simulink model "prodinvsys_ol"  (R2021b)
settings: Solver=ode15s  StartTime=0.0  StopTime=10.0  RelTol=1e-3  AbsTol=1e-6
values from neighbouring files (symbols this model uses):
  dchange = [60, 150]    [run_sim_ol.m]    (also in run_sim_spec.m = sim_spec.dchange; singlenodescm2022.m = input('Enter the demand change [2000 units]: '))
  rchange = [10, 1000]    [run_sim_ol.m]    (also in run_sim_spec.m = sim_spec.rchange; singlenodescm2022.m = input('Enter the inventory setpoint [20000 units]: '))
  thetaf = 20    [run_sim_ol.m]
  thetap = 10    [run_sim_ol.m]    (also in run_sim_spec.m = sim_spec.thetap; singlenodescm2022.m = input('Enter the production lead time (thetap) [10 time unit)
  thetas = 2    [run_sim_ol.m]    (also in run_sim_spec.m = sim_spec.thetas; singlenodescm2022.m = input('Enter the supply stream delivery time (thetad) [2 tim)
  Ts = 1    [run_sim_ol.m]
  vard = [85, 1000]    [run_sim_ol.m]    (also in run_sim_spec.m = sim_spec.vard; singlenodescm2022.m = input('Enter the unforecasted demand variance (vard) [1000]:)
settings Model: Creator=derivera  LastModifiedBy=billtubbs
settings SolverCC: AutoScaleAbsTol=off  AlgebraicLoopSolver=TrustRegion
settings DataIOCC: SaveFormat=Array  SignalLoggingSaveFormat=ModelDataLogs  ReturnWorkspaceOutputs=off
settings OptimizationCC: BooleanDataType=off  LifeSpan=inf
settings DebuggingCC: SaveWithParameterizedLinksMsg=none  UnderspecifiedInitializationDetection=Classic  MergeDetectMultiDrivingBlocksExec=none  SignalResolutionControl=TryResolveAllWithWarning  MultiTaskDSMMsg=warning  MultiTaskCondExecSysMsg=none  SFUnexpectedBacktrackingDiag=warning  SFNoUnconditionalDefaultTransitionDiag=warning  SFExecutionAtInitializationDiag=none  SFMachineParentedDataDiag=warning  ArithmeticOperatorsInVariantConditions=warning
settings HardwareCC: ProdBitPerPointer=32  ProdBitPerSizeT=32  ProdBitPerPtrDiffT=32  ProdLargestAtomicFloat=None  ProdIntDivRoundTo=Undefined  ProdEndianess=Unspecified  ProdWordSize=32  ProdHWDeviceType=32-bit Generic  TargetUnknown=on
settings ModelReferenceCC: PropagateSignalLabelsOutOfModel=off
settings SFSimCC: SimUseLocalCustomCode=off  CustomCodeUndefinedFunction=UseInterfaceOnly
settings RTWCC: RTWUseLocalCustomCode=off
settings CodeAppCC: StateflowObjectComments=on
settings GRTTargetCC: TargetLangStandard=C89/C90 (ANSI)  CombineOutputUpdateFcns=off  GRTInterface=on
settings ConfigComp: CovMetricSettings=dw  CovSaveCumulativeToWorkspaceVar=on  CovSaveSingleToWorkspaceVar=on  CovExternalEMLEnable=off  CovSFcnEnable=off

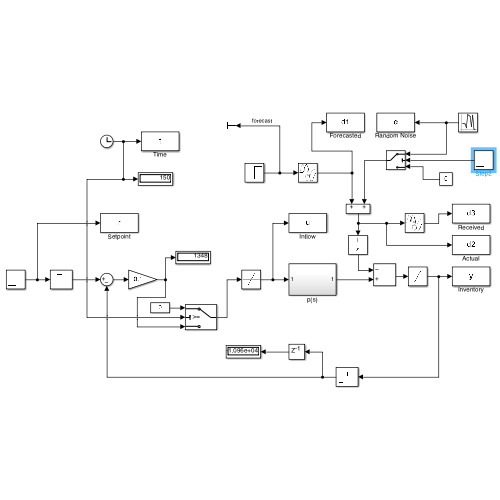
[thumbnail: Simulink's stored preview of the top-level diagram]
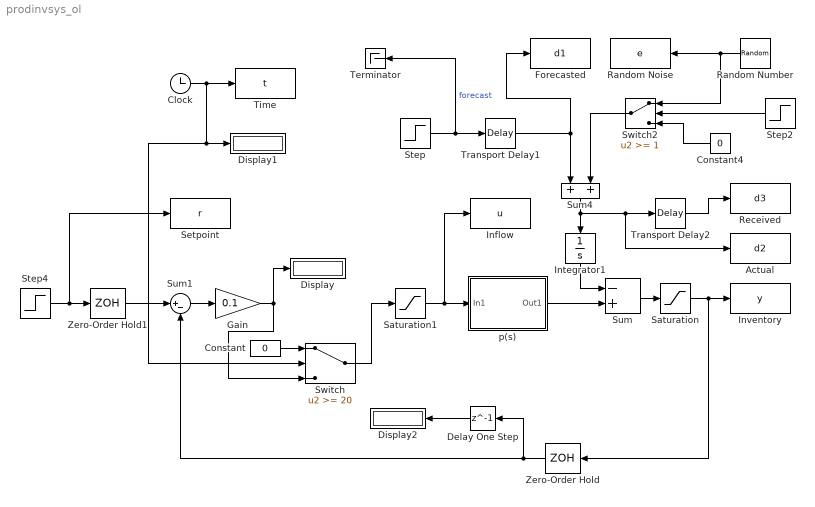
== system prodinvsys_ol ==
  Actual : ToWorkspace  VariableName=d2  SampleTime=Ts
  Clock : Clock
  Constant : Constant  Value=0
  Constant4 : Constant  Value=0
  Delay One Step : Delay  DelayLength=1
  Display : Display
  Display1 : Display
  Display2 : Display
  Forecasted : ToWorkspace  VariableName=d1  SampleTime=Ts
  Gain : Gain  Gain=0.1
  Inflow : ToWorkspace  VariableName=u  SampleTime=Ts
  Integrator1 : Integrator
  Inventory : ToWorkspace  VariableName=y  SampleTime=Ts
  Random Number : RandomNumber  Variance=vard(2)  SampleTime=1
  Random Noise : ToWorkspace  VariableName=e  SampleTime=Ts
  Received : ToWorkspace  VariableName=d3  SampleTime=Ts
  Saturation : Saturate  UpperLimit=inf  LowerLimit=-inf
  Saturation1 : Saturate  UpperLimit=inf  LowerLimit=-inf
  Setpoint : ToWorkspace  VariableName=r  SampleTime=Ts
  Step : Step  Time=dchange(1) - thetaf  After=dchange(2)  SampleTime=0
  Step2 : Step  Time=vard(1)  SampleTime=0
  Step4 : Step  Time=rchange(1)  After=rchange(2)  SampleTime=0
  Sum : Sum  Inputs=-+  InputSameDT=on  SaturateOnIntegerOverflow=on  OutDataTypeStr=Inherit: Same as first input
  Sum1 : Sum  Inputs=|+-
  Sum4 : Sum  InputSameDT=on  SaturateOnIntegerOverflow=on  OutDataTypeStr=Inherit: Same as first input
  Switch : Switch  Threshold=20
  Switch2 : Switch  Threshold=1  SaturateOnIntegerOverflow=on  InputSameDT=on
  Terminator : Terminator
  Time : ToWorkspace  VariableName=t  SampleTime=Ts
  Transport Delay1 : TransportDelay  DelayTime=thetaf
  Transport Delay2 : TransportDelay  DelayTime=thetas
  Zero-Order Hold : ZeroOrderHold  SampleTime=10
  Zero-Order Hold1 : ZeroOrderHold  SampleTime=10
  p(s) : Subsystem
  wires:
  p(s)/1(Out1) -> Sum/2
  Integrator1/1 -> Sum/1
  Sum/1 -> Saturation/1
  Saturation/1 -> Zero-Order Hold/1, Inventory/1
  Saturation1/1 -> Inflow/1, p(s)/1(In1)
  Step/1 -> Terminator/1, Transport Delay1/1  "forecast"
  Transport Delay2/1 -> Received/1
  Sum4/1 -> Transport Delay2/1, Actual/1, Integrator1/1
  Step2/1 -> Switch2/2
  Constant4/1 -> Switch2/3
  Switch2/1 -> Sum4/2
  Random Number/1 -> Random Noise/1, Switch2/1
  Clock/1 -> Switch/2, Display1/1, Time/1
  Sum1/1 -> Gain/1
  Step4/1 -> Setpoint/1, Zero-Order Hold1/1
  Zero-Order Hold/1 -> Delay One Step/1, Sum1/2
  Gain/1 -> Display/1, Switch/3
  Switch/1 -> Saturation1/1
  Constant/1 -> Switch/1
  Zero-Order Hold1/1 -> Sum1/1
  Transport Delay1/1 -> Sum4/1, Forecasted/1
  Delay One Step/1 -> Display2/1

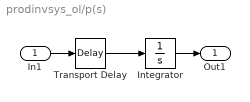
== system prodinvsys_ol/p(s) ==
  In1 : Inport
  Integrator : Integrator
  Transport Delay : TransportDelay  DelayTime=thetap
  Out1 : Outport  InitialOutput=0
  wires:
  Transport Delay/1 -> Integrator/1
  Integrator/1 -> Out1/1
  In1/1 -> Transport Delay/1
